simulink model "octocopter_control_flow"  (R2024a)
settings: Solver=FixedStepAuto  StartTime=0.0  StopTime=inf
model workspace (MAT data in the model file):
  Ixx_values = 1.545e-05
  Iyy_values = 0.00073574
  Izz_values = 0.00074861
  base_link_Ixx = 7.46
  base_link_Iyy = 1.52
  base_link_Izz = 8.88
  base_link_mass = 19.0939
  gps0_Ixx = 2.1733e-06
  gps0_Iyy = 2.1733e-06
  gps0_Izz = 1.8e-07
  gps0_mass = 0.01
  i = 8
  imu_link_Ixx = 1e-05
  imu_link_Iyy = 1e-05
  imu_link_Izz = 1e-05
  imu_link_mass = 0.015
  masses = 0.085251
  phi = sym
  phi.s = 'symobj::fromString("eJytVL1OwzAQdpqWPwkhoaJCp0jwBIydCoKBEYoYWCyHmGLkOCXnlGbjKXgneCpst6LONQ0MjfTJzt35u+/uLIeEkBYhH59mbYdBxyzDPpl/odl3F3sTQ3YtoAQGIMbKmSv+c4t3LvIkmrJcsFjySLGUQ1QATyKhIijTLH69KtK0vEm40uJZ8Jz4OVuIs23xksnE2HteTL9mj/W6syAzjexbFqATKWKXe48sv30L4HpUphdSMOAwr/PEy/HtxQeIe9tiAoI+MFvY8MzTebo84/79vAcWc02DwfVskpmO4Vl8efFt9N9BfE6Hx+P7QgujEfOv1EF/J13xHVmsHeWSs1M7jyIGpP2wQYebFeVvBZPkr3429crn3LGATE65uwGV3jjfJQPxNOIa8fRQrKsn51ZZhd/hjlZ6gTV1US2+77hulkJpPnYdXs31uLlcrv6caZGp+rpu6eYejP9epKZHofniCJXw2UpeVyQ1iZkC6j0sliP0mhFEixXbgzX2+8X6AxDlhOk=", 2)'
  phi.Digits = 32
  rotors(1).mass = 0.085251
  rotors(1).Ixx = 1.545e-05
  rotors(1).Iyy = 0.00073574
  rotors(1).Izz = 0.00074861
  rotors(2).mass = 0.085251
  rotors(2).Ixx = 1.545e-05
  rotors(2).Iyy = 0.00073574
  rotors(2).Izz = 0.00074861
  rotors(3).mass = 0.085251
  rotors(3).Ixx = 1.545e-05
  rotors(3).Iyy = 0.00073574
  rotors(3).Izz = 0.00074861
  rotors(4).mass = 0.085251
  rotors(4).Ixx = 1.545e-05
  rotors(4).Iyy = 0.00073574
  rotors(4).Izz = 0.00074861
  rotors(5).mass = 0.085251
  rotors(5).Ixx = 1.545e-05
  rotors(5).Iyy = 0.00073574
  rotors(5).Izz = 0.00074861
  rotors(6).mass = 0.085251
  rotors(6).Ixx = 1.545e-05
  rotors(6).Iyy = 0.00073574
  rotors(6).Izz = 0.00074861
  rotors(7).mass = 0.085251
  rotors(7).Ixx = 1.545e-05
  rotors(7).Iyy = 0.00073574
  rotors(7).Izz = 0.00074861
  rotors(8).mass = 0.085251
  rotors(8).Ixx = 1.545e-05
  rotors(8).Iyy = 0.00073574
  rotors(8).Izz = 0.00074861
  theta = sym
  theta.s = 'symobj::fromString("eJytVL1OwzAQdpqWPwkhoaJCp0jwBIydCoKBESoxsFgOOYqR45ScU5qNp+CdylNhuxV13DQwNNInO3fn7767sxwSQlqEfH7ptR0GHb0M+2TxhXrfXe51DNk3wBIZIh9La674Lw0+gOdJNGU5Z7GASLIUMCoQkojLCMs0i99uijQt7xKQir9wyImbs+Vxtg1eM5Foe8+J6dfsfb32LIpMefYdA1SJ4LHNfUBW36EBghqV6ZXgDAEXdZ45Ob6d+MDj3jWYIKePzBQ2vHB0nq/O2H8375HBQtNgcDubZLpj/izmTnzb++94fFaHw+P6QgOt0edfq4P+TrriOzHYOMoVZ6d2HkWMnvbjBh12VhTeCybIX/1s6pXLuWeAmZiCvQGV3ljfNUP+PALl8fS8WFtPDkZZhd/igVZ64WvqerW4vtO6WXKpYGw7vJ7raXu5bP05UzyT9XXd0+09GP+9SE2PQvPF4TKB2VpeWyTViZlE6jwshiN0mhFEy9W3BxvssFx/ABFthPo=", 2)'
  theta.Digits = 32
  total_Ixx = 7.46
  total_Iyy = 1.53
  total_Izz = 8.89
  total_mass = 20
  total_rotor_Ixx = 0.0001236
  total_rotor_Iyy = 0.00588592
  total_rotor_Izz = 0.00598888
  total_rotor_masses = 0.682008
  u = sym
  u.s = 'symobj::fromString("eJytVL1OwzAQdpqWPwkhoaJCp0jwBIydCoKBESoxsFgOOYqR45ScU5qNp+CdylNhuxV13DQwNNInO3fn7767sxwSQlqEfH7ptR0GHb0M+2TxhXrfXe51DNk3wBIZIh9La674Lw0+gOdJNGU5Z7GASLIUMCoQkojLCMs0i99uijQt7xKQir9wyImbs+Vxtg1eM5Foe8+J6dfsfb32LIpMefYdA1SJ4LHNfUBW36EBghqV6ZXgDAEXdZ45Ob6d+MDj3jWYIKePzBQ2vHB0nq/O2H8375HBQtNgcDubZLpj/izmTnzb++94fFaHw+P6QgOt0edfq4P+TrriOzHYOMoVZ6d2HkWMnvbjBh12VhTeCybIX/1s6pXLuWeAmZiCvQGV3ljfNUP+PALl8fS8WFtPDkZZhd/igVZ64WvqerW4vtO6WXKpYGw7vJ7raXu5bP05UzyT9XXd0+09GP+9SE2PQvPF4TKB2VpeWyTViZlE6jwshiN0mhFEy9W3Bxvs0+X6AxH1hQs=", 2)'
  u.Digits = 32
  v = sym
  v.s = 'symobj::fromString("eJytVL1OwzAQdpqWPwkhoaJCp0jwBIydCoKBESoxsFgOOYqR45ScU5qNjTfgneCpsN2KOm4aGBrpk52783ff3VkOCSEtQt4/9doOg45ehn0y/0K97y72OobsGmCJDJGPpTVX/OcGb8DzJJqynLNYQCRZChgVCEnEZYRlmsUvV0WaljcJSMWfOOTEzdnyONsGz5lItL3nxPRr9r5eexZFpjz7lgGqRPDY5t4jy2/fAEGNyvRCcIaA8zpPnBzfTnzgcW8bTJDTe2YKG545Ok+XZ+y/m/fAYK5pMLieTTLdMX8WX0582/vveHxWh8Pj+kIDrdHnX6mD/k664jsyWDvKJWendh5FjJ72wwYddlYUXgsmyF/9bOqVy7ljgJmYgr0Bld5Y3yVD/jgC5fH0vFhbTw5GWYXf4o5WeuFr6nq1uL7jullyqWBsO7ya62FzuWz9OVM8k/V13dLNPRj/vUhNj0LzxeEygdlKXlsk1YmZROo8LIYjdJoRRIvVtwdr7B+L9QcSfYUc", 2)'
  v.Digits = 32
  w = sym
  w.s = 'symobj::fromString("eJytVL1OwzAQdpqWPwkhoaJCp0jwBIydCoKBESoxsFgOOYqR45ScU5qNp0C8EjwVtltRx00DQyN9snN3/u67O8shIaRFyPuHXtth0NHLsE/mX6j33cVex5BdAyyRIfKxtOaK/9zgDXieRFOWcxYLiCRLAaMCIYm4jLBMs/jlqkjT8iYBqfgTh5y4OVseZ9vgOROJtvecmH7N3tdrz6LIlGffMkCVCB7b3Htk+e0bIKhRmV4IzhBwXueJk+PbiQ887m2DCXJ6z0xhwzNH5+nyjP138x4YzDUNBtezSaY75s/iy4lve/8dj8/qcHhcX2igNfr8K3XQ30lXfEcGa0e55OzUzqOI0dN+2KDDzorCa8EE+aufTb1yOXcMMBNTsDeg0hvru2TIH0egPJ6eF2vrycEoq/Bb3NFKL3xNXa8W13dcN0suFYxth1dzPWwul60/Z4pnsr6uW7q5B+O/F6npUWi+OFwmMFvJa4ukOjGTSJ2HxXCETjOCaLH69mCN/XOx/gATBYUt", 2)'
  w.Digits = 32
  x = sym
  x.s = 'symobj::fromString("eJytVEtOwzAQdZqWn4SQUFGhq0hwApZdFQQLllCJBRvLIUMxcpyScUqz4xTcgaPAqbDdijpuGlg00pOdmfGbNzOWQ0JIi5D3D722w6Cjl2GfzL9Q77uLvY4huwZYIkPkY2nNFf+5wRvwPImmLOcsFhBJlgJGBUIScRlhmWbxy1WRpuVNAlLxJw45cXO2PM62wXMmEm3vOTH9mr2v155FkSnPvmWAKhE8trn3yPLbN0BQozK9EJwh4LzOEyfHtxMfeNzbBhPk9J6ZwoZnjs7T5Rn77+Y9MJhrGgyuZ5NMd8yfxZcT3/b+Ox6f1eHwuL7QQGv0+VfqoL+TrviODNaOcsnZqZ1HEaOn/bBBh50VhdeCCfJXP5t65XLuGGAmpmBvQKU31nfJkD+OQHk8PS/W1pODUVbht7ijlV74mrpeLa7vuG6WXCoY2w6v5nrYXC5bf84Uz2R9Xbd0cw/Gfy9S06PQfHG4TGC2ktcWSXViJpE6D4vhCJ1mBNFi9e3BGvvnYv0BE42FPg==", 2)'
  x.Digits = 32
  y = sym
  y.s = 'symobj::fromString("eJytVEtOwzAQdZqWn4SQUFGhq0hwApZdFQQLllCJBRvLIUMxcpyScUqz4xQchhvAqbDdijpuGlg00pOdmfGbNzOWQ0JIi5D3D722w6Cjl2GfzL9Q77uLvY4huwZYIkPkY2nNFf+5wRvwPImmLOcsFhBJlgJGBUIScRlhmWbxy1WRpuVNAlLxJw45cXO2PM62wXMmEm3vOTH9mr2v155FkSnPvmWAKhE8trn3yPLbN0BQozK9EJwh4LzOEyfHtxMfeNzbBhPk9J6ZwoZnjs7T5Rn77+Y9MJhrGgyuZ5NMd8yfxZcT3/b+Ox6f1eHwuL7QQGv0+VfqoL+TrviODNaOcsnZqZ1HEaOn/bBBh50VhdeCCfJXP5t65XLuGGAmpmBvQKU31nfJkD+OQHk8PS/W1pODUVbht7ijlV74mrpeLa7vuG6WXCoY2w6v5nrYXC5bf84Uz2R9Xbd0cw/Gfy9S06PQfHG4TGC2ktcWSXViJpE6D4vhCJ1mBNFi9e3BGvvnYv0BFBWFTw==", 2)'
  y.Digits = 32
  z = sym
  z.s = 'symobj::fromString("eJytVL1OwzAQdpqWPwkhoaJCp0jwBIydCoKBESoxsFgOOYqR45ScU5qNp+CdgJfCdivquGlgaKRPdu7O3313ZzkkhLQIef/QazsMOnoZ9sn8C/W+u9jrGLJrgCUyRD6W1lzxnxu8Ac+TaMpyzmIBkWQpYFQgJBGXEZZpFr9cFWla3iQgFX/ikBM3Z8vjbBs8ZyLR9p4T06/Z+3rtWRSZ8uxbBqgSwWObe48sv30DBDUq0wvBGQLO6zxxcnw58YHHvW0wQU7vmSlseOboPF2esf9u3gODuabB4Ho2yXTH/Fl8OvFt77/j8VkdDo/rCw20Rp9/pQ76O+mK78hg7SiXnJ3aeRQxetoPG3TYWVF4LZggf/WzqVcu544BZmIK9gZUemN9lwz54wiUx9PzYm09ORhlFX6LO1rpha+p69Xi+o7rZsmlgrHt8Gquh83lsvXnTPFM1td1Szf3YPz3IjU9Cs0Xh8sEZit5bZFUJ2YSqfOwGI7QaUYQLVbfHqyxfy/WHxSdhWA=", 2)'
  z.Digits = 32
values from neighbouring files (symbols this model uses):
  err1Enable = 0    [drone_6dof.m]    (also in octocopter_model_for_agressive.m; octocopter_model_for_orbit.m)
  err2Enable = 0    [drone_6dof.m]    (also in octocopter_model_for_agressive.m; octocopter_model_for_orbit.m)
  err3Enable = 0    [drone_6dof.m]    (also in octocopter_model_for_agressive.m; octocopter_model_for_orbit.m)
  err4Enable = 0    [drone_6dof.m]    (also in octocopter_model_for_agressive.m; octocopter_model_for_orbit.m)
  err5Enable = 0    [drone_6dof.m]    (also in octocopter_model_for_agressive.m; octocopter_model_for_orbit.m)
  err6Enable = 0    [drone_6dof.m]    (also in octocopter_model_for_agressive.m; octocopter_model_for_orbit.m)
  err7Enable = 0    [drone_6dof.m]    (also in octocopter_model_for_agressive.m; octocopter_model_for_orbit.m)
  err8Enable = 0    [drone_6dof.m]    (also in octocopter_model_for_agressive.m; octocopter_model_for_orbit.m)
  EulerInt_initial = [0;0;0]    [drone_6dof.m]    (also in octocopter_model_for_agressive.m; octocopter_model_for_orbit.m)
  motorErr1Time = 0    [drone_6dof.m]    (also in octocopter_model_for_agressive.m; octocopter_model_for_orbit.m)
  motorErr2Time = 0    [drone_6dof.m]    (also in octocopter_model_for_agressive.m; octocopter_model_for_orbit.m)
  motorErr3Time = 0    [drone_6dof.m]    (also in octocopter_model_for_agressive.m; octocopter_model_for_orbit.m)
  motorErr4Time = 0    [drone_6dof.m]    (also in octocopter_model_for_agressive.m; octocopter_model_for_orbit.m)
  motorErr5Time = 0    [drone_6dof.m]    (also in octocopter_model_for_agressive.m; octocopter_model_for_orbit.m)
  motorErr6Time = 0    [drone_6dof.m]    (also in octocopter_model_for_agressive.m; octocopter_model_for_orbit.m)
  motorErr7Time = 0    [drone_6dof.m]    (also in octocopter_model_for_agressive.m; octocopter_model_for_orbit.m)
  motorErr8Time = 0    [drone_6dof.m]    (also in octocopter_model_for_agressive.m; octocopter_model_for_orbit.m)
  omegaInt_initial = [0;0;0]    [drone_6dof.m]    (also in octocopter_model_for_agressive.m; octocopter_model_for_orbit.m)
  PosInertialInt_initial = [0;0;0]    [drone_6dof.m]    (also in octocopter_model_for_agressive.m; octocopter_model_for_orbit.m)
  vbInt_initial = [0;0;0]    [drone_6dof.m]    (also in octocopter_model_for_agressive.m; octocopter_model_for_orbit.m)
undefined symbols (not defined in the file or in its folder): DiscIntNeverNeededParam, PID_x_D, PID_x_I, PID_x_N, PID_y_D, PID_y_I, PID_y_N, PID_z_D, PID_z_I, PID_z_N, rad, rotor_max_rad_per_s, rotor_min_rad_per_s, s
libraries: robotlib x15, slpidlib x10, aerolibconvert2 x10, cstblocks x7, simulink x6, sharedtransform x4, dspmathops x1, vrlib x1, sharedutil x1, simulink_extras x1
(part 1 of 2)
settings Model: PacingRate=10  Creator=hmcl  LastModifiedBy=hmcl
settings RTWCC: GPUComputeCapability=3.5

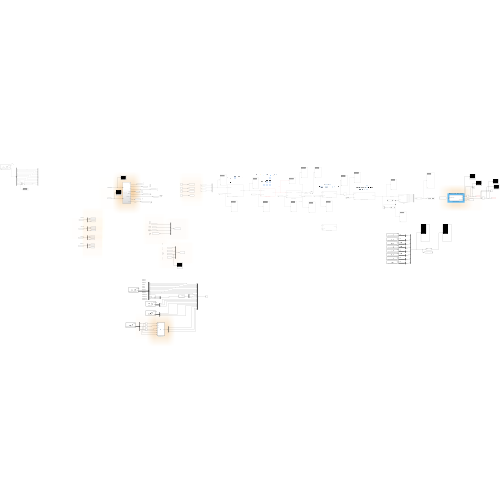
[thumbnail: Simulink's stored preview of the top-level diagram]
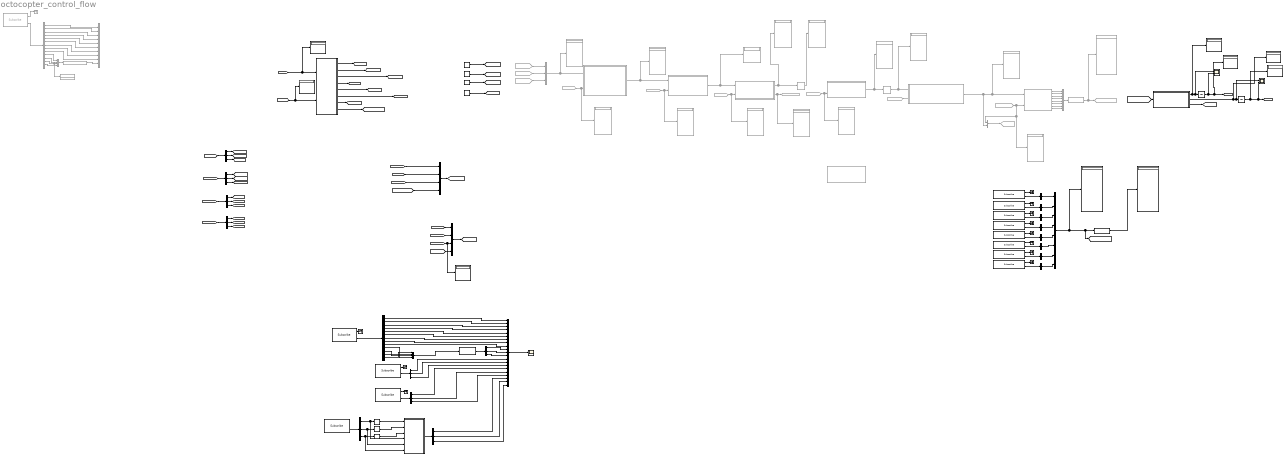
== system octocopter_control_flow ==
  note: Position.X,
      | Position.Y,
      | Position.Z,
      | Linear.X
      | Linear.Y
      | Linear.Z
      | Angular.X
      | Angular.Y
      | Angular.Z
      | Orientation.X,
      | Orientation.Y,
      | Orientation.Z,
      | Orientation.W,
  note: earth frame
  note: phi_dot
      | theta_dot
      | psi_dot
  note: x_dot
      | y_dot
      | z_dot
  note: phi
      | theta
      | psi
  note: u
      | v
      | w
  note: p
      | q
      | r
  note: p_dot
      | q_dot
      | r_dot
  note: u_dot
      | v_dot
      | w_dot
  note: x
      | y
      | z
  note: earth frame
  note: earth frame
  note: earth frame
  note: Motor Force and Torque
  note: u_dot
      | v_dot
      | w_dot
  note: x_dot
      | y_dot
      | z_dot
  note: phi_dot
      | theta_dot
      | psi_dot
  note: p_dot
      | q_dot
      | r_dot
  note: phi
      | theta
      | psi
  note: p
      | q
      | r
  note: x
      | y
      | z
  note: u
      | v
      | w
  Angular Rate Controller : Subsystem  Commented=on  mask{MC_ROLLRATE_K=0.01, MC_ROLLRATE_P=0.044, MC_ROLLRATE_I=0.05, MC_ROLLRATE_D=0.0012, MC_RR_INT_LIM=1000, MC_PITCHRATE_K=0.01, MC_PITCHRATE_P=0.044, MC_PITCHRATE_I=0.05, MC_PITCHRATE_D=0.0012, MC_PR_INT_LIM=1000, MC_YAWRATE_K=0.01, MC_YAWRATE_P=0.044, MC_YAWRATE_I=0.05, MC_YAWRATE_D=0.0012, MC_YR_INT_LIM=1000, IMU_DGYRO_CUTOFF=30, IMU_GYRO_CUTOFF=40}
      mask prompts: MC_ROLLRATE_K "MC_ROLLRATE_K ="; MC_ROLLRATE_P "MC_ROLLRATE_P ="; MC_ROLLRATE_I "MC_ROLLRATE_I ="; MC_ROLLRATE_D "MC_ROLLRATE_D ="; MC_RR_INT_LIM "MC_RR_INT_LIM ="; MC_PITCHRATE_K "MC_PITCHRATE_K ="; MC_PITCHRATE_P "MC_PITCHRATE_P ="; MC_PITCHRATE_I "MC_PITCHRATE_I ="; MC_PITCHRATE_D "MC_PITCHRATE_D ="; MC_PR_INT_LIM "MC_PR_INT_LIM ="; MC_YAWRATE_K "MC_YAWRATE_K ="; MC_YAWRATE_P "MC_YAWRATE_P ="; MC_YAWRATE_I "MC_YAWRATE_I ="; MC_YAWRATE_D "MC_YAWRATE_D ="; MC_YR_INT_LIM "MC_YR_INT_LIM ="; IMU_DGYRO_CUTOFF "IMU_DGYRO_CUTOFF ="; IMU_GYRO_CUTOFF "IMU_GYRO_CUTOFF ="
      mask DialogControl DescTextVar Prompt: Angular rate controller, based on PX4 architecture
      mask DialogControl ROLL Prompt: Roll
      mask DialogControl PITCH Prompt: Pitch
      mask DialogControl YAW Prompt: Yaw
  Angular Velocity Conversion : aerolibconvert2/Angular Velocity Conversion  Commented=on  IU=rad/s  OU=rpm
  Angular Velocity Conversion1 : aerolibconvert2/Angular Velocity Conversion  IU=rad/s  OU=rpm
  Attitude Controller : Subsystem  Commented=on  mask{MC_ROLL_P=4, MC_PITCH_P=4, MC_YAW_P=4, MC_ROLLRATE_MAX=10, MC_PITCHRATE_MAX=10, MC_YAWRATE_MAX=10, MC_ACRO_R_MAX=2, MC_YAW_WEIGHT=0.1}
      mask prompts: MC_ROLL_P "MC_ROLL_P ="; MC_PITCH_P "MC_PITCH_P ="; MC_YAW_P "MC_YAW_P ="; MC_ROLLRATE_MAX "MC_ROLLRATE_MAX ="; MC_PITCHRATE_MAX "MC_PITCHRATE_MAX ="; MC_YAWRATE_MAX "MC_YAWRATE_MAX ="; MC_ACRO_R_MAX "MC_ACRO_R_MAX ="; MC_YAW_WEIGHT "MC_YAW_WEIGHT ="
      mask DialogControl DescTextVar Prompt: Attitude Controller - based on PX4 architecture
  Attitude Controller1 : Subsystem  Commented=on  mask{MC_ROLL_P=6.5, MC_PITCH_P=6.5, MC_YAW_P=2.8, MC_ROLLRATE_MAX=220, MC_PITCHRATE_MAX=220, MC_YAWRATE_MAX=200, MC_ACRO_R_MAX=100, MC_YAW_WEIGHT=0.4}
      mask prompts: MC_ROLL_P "MC_ROLL_P ="; MC_PITCH_P "MC_PITCH_P ="; MC_YAW_P "MC_YAW_P ="; MC_ROLLRATE_MAX "MC_ROLLRATE_MAX ="; MC_PITCHRATE_MAX "MC_PITCHRATE_MAX ="; MC_YAWRATE_MAX "MC_YAWRATE_MAX ="; MC_ACRO_R_MAX "MC_ACRO_R_MAX ="; MC_YAW_WEIGHT "MC_YAW_WEIGHT ="
      mask DialogControl DescTextVar Prompt: Attitude Controller - based on PX4 architecture
  Bus Selector{,3..9} (8 alike) : BusSelector  OutputSignals=Data
  Bus Selector1 : BusSelector  OutputSignals=Pose.Pose.Position.X,Pose.Pose.Position.Y,Pose.Pose.Position.Z,Twist.Twist.Linear.X,Twist.Twist.Linear.Y,Twist.Twist.Linear.Z,Twist.Twist.Angular.X,Twist.Twist.Angular.Y,Twist.Twist.Angular.Z,Pose.Pose.Orientation.X,Pose.Pose.Orientation.Y,Pose.Pose.Orientation.Z,Pose.Pose.Orientation.W
  Bus Selector10 : BusSelector  OutputSignals=X,Y,Z
  Bus Selector11 : BusSelector  OutputSignals=X,Y,Z
  Bus Selector12 : BusSelector  OutputSignals=Twist.Twist.Angular.X,Twist.Twist.Angular.Y,Twist.Twist.Angular.Z
  Bus Selector2 : BusSelector  Commented=on  OutputSignals=Pose.Pose.Position.X,Pose.Pose.Position.Y,Pose.Pose.Position.Z,Twist.Twist.Linear.X,Twist.Twist.Linear.Y,Twist.Twist.Linear.Z,Twist.Twist.Angular.X,Twist.Twist.Angular.Y,Twist.Twist.Angular.Z,Pose.Pose.Orientation.X,Pose.Pose.Orientation.Y,Pose.Pose.Orientation.Z,Pose.Pose.Orientation.W
  Constant : Constant  Value=0
  Constant1 : Constant  Value=0
  Constant2 : Constant  Value=10
  Constant3 : Constant  Value=0
  ControlMatrixAllocation Mixer : Subsystem  Commented=on  mask{Ct=5.781e-06, Cq=1.839e-07, L1=0.545, L2=0.36, L3=1.08}
      mask prompts: Ct "Ct ="; Cq "Cq ="; L1 "L1 ="; L2 "L2 ="; L3 "L3 ="
  Demux{,1..5} (6 alike) : Demux  Outputs=3
  Derivative : Derivative
  Derivative1 : Derivative
  Derivative2 : Derivative
  Display{,1..2,10,12..23} (16 alike) : Display  Commented=on
  Display{3..9,24..25} (9 alike) : Display
  From : From  Commented=on  GotoTag=zRef
  From1 : From  Commented=on  GotoTag=yRef
  From10 : From  Commented=on  GotoTag=phithetapsi
  From11 : From  Commented=on  GotoTag=OMEGA
  From12 : From  Commented=on  GotoTag=desired_Thrust
  From2 : From  Commented=on  GotoTag=xRef
  From7 : From  Commented=on  GotoTag=xyz
  From8 : From  Commented=on  GotoTag=V
  From9 : From  Commented=on  GotoTag=desired_yaw
  Goto13 : Goto  Commented=on  GotoTag=desired_Thrust
  Goto25 : Goto  Commented=on  GotoTag=omegaMotorSpeed
  Goto32 : Goto  Commented=on  GotoTag=desired_input
  Inertial to Body : Subsystem  Commented=on  mask{m=total_mass}
      mask prompts: m "m ="
      mask DialogControl DescTextVar Prompt: Acceleration and yaw to attitude Controller - based on PX4 architecture
  MATLAB Function : MATLAB Function  TreatAsAtomicUnit=on
  MotorForceCalculation : Subsystem  mask{Ct=6.5, Cq=-0.325, L1=0.545, L2=0.36, L3=1.08}
      mask prompts: Ct "Ct ="; Cq "Cq ="; L1 "L1 ="; L2 "L2 ="; L3 "L3 ="
  Mux : Mux  Commented=on  Inputs=3
  Mux1 : Mux  Commented=on  Inputs=8
  Mux2 : Mux  Commented=on  Inputs=10
  Mux3 : Mux
  Mux4 : Mux
  Mux5 : Mux  Inputs=21
  Mux6 : Mux  Commented=on
  Mux7 : Mux
  Mux8 : Mux  Commented=on  Inputs=2
  Mux9 : Mux  Inputs=8
  Position Controller : Subsystem  Commented=on  mask{MPC_XY_P=1, MPC_XY_VEL_ALL=10, MPC_Z_P=1, MPC_Z_VEL_ALL=100}
      mask prompts: MPC_XY_P "MPC_XY_P ="; MPC_XY_VEL_ALL "MPC_XY_VEL_ALL ="; MPC_Z_P "MPC_Z_P ="; MPC_Z_VEL_ALL "MPC_Z_VEL_ALL ="
      mask DialogControl DescTextVar Prompt: Position Controller - based on PX4 architecture
  Quaternions to Rodrigues1 : Quat2Rod  Commented=on
  Quaternions to Rotation Angles : sharedtransform/Quaternions to Rotation Angles  rotationOrder=ZYX  aMode=aMode
  Rate Transition2 : RateTransition  Commented=on  OutPortSampleTime=1/1000
  Rate Transition5 : RateTransition  Commented=on  OutPortSampleTime=1/1000
  Scope : Scope  NumInputPorts=2
  Scope1 : Scope  NumInputPorts=2
  Scope2 : Scope
  Subscribe : robotlib/Subscribe  topicSource=Select from ROS network  topic=/my/octocopter3/motor_speed/0  messageType=std_msgs/Float64  SampleTime=-1  legacyBusStruct=off  messageQueueLength=1
  Subscribe1 : robotlib/Subscribe  topicSource=Select from ROS network  topic=/mavros/local_position/odom  messageType=nav_msgs/Odometry  SampleTime=-1  legacyBusStruct=off  messageQueueLength=1
  Subscribe10 : robotlib/Subscribe  topicSource=Select from ROS network  topic=/thrust_vector  messageType=geometry_msgs/Vector3  SampleTime=-1  legacyBusStruct=off  messageQueueLength=1
  Subscribe11 : robotlib/Subscribe  topicSource=Select from ROS network  topic=/torque_vector  messageType=geometry_msgs/Vector3  SampleTime=-1  legacyBusStruct=off  messageQueueLength=1
  Subscribe12 : robotlib/Subscribe  topicSource=Select from ROS network  topic=/mavros/local_position/odom  messageType=nav_msgs/Odometry  SampleTime=-1  legacyBusStruct=off  messageQueueLength=1
  Subscribe2 : robotlib/Subscribe  Commented=on  topicSource=Select from ROS network  topic=/mavros/local_position/odom  messageType=nav_msgs/Odometry  SampleTime=-1  legacyBusStruct=off  messageQueueLength=1
  Subscribe3 : robotlib/Subscribe  topicSource=Select from ROS network  topic=/my/octocopter3/motor_speed/1  messageType=std_msgs/Float64  SampleTime=-1  legacyBusStruct=off  messageQueueLength=1
  Subscribe4 : robotlib/Subscribe  topicSource=Select from ROS network  topic=/my/octocopter3/motor_speed/2  messageType=std_msgs/Float64  SampleTime=-1  legacyBusStruct=off  messageQueueLength=1
  Subscribe5 : robotlib/Subscribe  topicSource=Select from ROS network  topic=/my/octocopter3/motor_speed/3  messageType=std_msgs/Float64  SampleTime=-1  legacyBusStruct=off  messageQueueLength=1
  Subscribe6 : robotlib/Subscribe  topicSource=Select from ROS network  topic=/my/octocopter3/motor_speed/4  messageType=std_msgs/Float64  SampleTime=-1  legacyBusStruct=off  messageQueueLength=1
  Subscribe7 : robotlib/Subscribe  topicSource=Select from ROS network  topic=/my/octocopter3/motor_speed/5  messageType=std_msgs/Float64  SampleTime=-1  legacyBusStruct=off  messageQueueLength=1
  Subscribe8 : robotlib/Subscribe  topicSource=Select from ROS network  topic=/my/octocopter3/motor_speed/6  messageType=std_msgs/Float64  SampleTime=-1  legacyBusStruct=off  messageQueueLength=1
  Subscribe9 : robotlib/Subscribe  topicSource=Select from ROS network  topic=/my/octocopter3/motor_speed/7  messageType=std_msgs/Float64  SampleTime=-1  legacyBusStruct=off  messageQueueLength=1
  Subsystem : Subsystem
  Terminator{,1..10} (11 alike) : Terminator
  Terminator12 : Terminator  Commented=on
  Unit Delay : UnitDelay  SampleTime=-1  HasFrameUpgradeWarning=on
  Unit Delay1 : UnitDelay  SampleTime=-1  HasFrameUpgradeWarning=on
  Velocity Controller : Subsystem  Commented=on  mask{MPC_XY_VEL_P_ACC=1, MPC_XY_VEL_I_ACC=0.1, MPC_XY_VEL_D_ACC=0.01, MPC_Z_VEL_P_ACC=1, MPC_Z_VEL_I_ACC=0.1, MPC_Z_VEL_D_ACC=0.01, MPC_VELD_LP=5.0, MPC_TILTMAX_AIR=45, MPC_THR_MAX=1000}
      mask prompts: MPC_XY_VEL_P_ACC "MPC_XY_VEL_P_ACC ="; MPC_XY_VEL_I_ACC "MPC_XY_VEL_I_ACC ="; MPC_XY_VEL_D_ACC "MPC_XY_VEL_D_ACC ="; MPC_Z_VEL_P_ACC "MPC_Z_VEL_P_ACC ="; MPC_Z_VEL_I_ACC "MPC_Z_VEL_I_ACC ="; MPC_Z_VEL_D_ACC "MPC_Z_VEL_D_ACC ="; MPC_VELD_LP "MPC_VELD_LP ="; MPC_TILTMAX_AIR "MPC_TILTMAX_AIR ="; MPC_THR_MAX "MPC_THR_MAX ="
      mask DialogControl DescTextVar Prompt: Velocity Controller - based on PX4 architecture
      mask DialogControl Container3 Prompt: XY -  Velocity
      mask DialogControl Container4 Prompt: Z - Velocity
      mask DialogControl Container5 Prompt: General Parameters
  wires:
  Quaternions to Rodrigues1/1 -> Mux2/10
  Bus Selector2/4 -> Mux2/4  "<X>"
  Bus Selector2/10 -> Mux6/1  "<X>"
  Bus Selector2/3 -> Mux2/3  "<Z>"
  Bus Selector2/7 -> Mux2/7  "<X>"
  Bus Selector2/8 -> Mux2/8  "<Y>"
  Bus Selector2/1 -> Mux2/1  "<X>"
  Bus Selector2/9 -> Mux2/9  "<Z>"
  Mux6/1 -> Quaternions to Rodrigues1/1
  Subscribe2/2 -> Bus Selector2/1
  Bus Selector2/6 -> Mux2/6  "<Z>"
  Bus Selector2/12 -> Mux6/3, Display1/1  "<Z>"
  Bus Selector2/11 -> Mux6/2  "<Y>"
  Bus Selector2/5 -> Mux2/5  "<Y>"
  Bus Selector2/2 -> Mux2/2  "<Y>"
  Bus Selector2/13 -> Mux6/4  "<W>"
  Subscribe2/1 -> Terminator12/1
  Subsystem/1(xyz) -> [xyz]
  Subsystem/2(V) -> [V]  "V"
  Subsystem/4(VB_dot) -> [VB_dot]  "VB_dot"
  Subsystem/5(phithetapsi) -> [phithetapsi]
  Subsystem/8(pqr_dot) -> [OMEGAB_dot]  "pqr_dot"
  Subsystem/7(pqr) -> [OMEGAB]  "pqr"
  Subsystem/3(VB) -> [VB]  "VB"
  Subsystem/6(phithetapsi_dot) -> [OMEGA]
  [xyz] -> Demux/1
  [V] -> Demux1/1
  [phithetapsi] -> Demux2/1
  [OMEGA] -> Demux3/1
  Demux2/1 -> [phi]
  Demux2/2 -> [theta]
  Demux2/3 -> [psi]
  Demux3/1 -> [phidot]
  Demux3/2 -> [thetadot]
  Demux3/3 -> [psidot]
  Demux/3 -> [z]
  Demux/1 -> [x]
  Demux/2 -> [y]
  Demux1/1 -> [x_dot]
  Demux1/2 -> [y_dot]
  Demux1/3 -> [z_dot]
  From7/1 -> Display13/1, Position Controller/2(Current position)  "xyz"
  From2/1 -> Mux/1
  From1/1 -> Mux/2
  From/1 -> Mux/3
  Mux/1 -> Display12/1, Position Controller/1(Setpoint position)
  Velocity Controller/1(Acc S.P) -> Display2/1, Inertial to Body/1(Setpoints acceleration)  "Acc S.P"
  From9/1 -> Display15/1, Inertial to Body/2(Yaw.SP)
  Inertial to Body/1(quat_attitude_sp) -> Display16/1, Rate Transition2/1  "attitude qutanion value"
  Inertial to Body/2(Thrust) -> Display22/1, Goto13/1  "desired thrust"
  Rate Transition2/1 -> Display17/1
  From10/1 -> Display23/1, Attitude Controller/2(Orientation)  "phithetapsi"
  Attitude Controller/1(S.P Rates) -> Display18/1, Rate Transition5/1  "S.P Rates"
  Rate Transition5/1 -> Display19/1, Angular Rate Controller/1(rates s.p)
  From11/1 -> Angular Rate Controller/2(Gyro)
  Angular Rate Controller/1(Delta S.P) -> Mux8/2, Display20/1, ControlMatrixAllocation Mixer/1(Tau_roll,pitch,yaw)  "desired_torque"
  From12/1 -> Mux8/1, Display21/1, ControlMatrixAllocation Mixer/2(Thrust)  "desire_thrust"
  Constant/1 -> [xRef]
  Constant2/1 -> [zRef]
  Constant1/1 -> [yRef]
  Constant3/1 -> [desired_yaw]
  ControlMatrixAllocation Mixer/1(Omega 1) -> Mux1/1
  ControlMatrixAllocation Mixer/2(Omega 2) -> Mux1/2
  ControlMatrixAllocation Mixer/3(Omega 3) -> Mux1/3
  ControlMatrixAllocation Mixer/4(Omega 4) -> Mux1/4
  ControlMatrixAllocation Mixer/5(Omega 5) -> Mux1/5
  ControlMatrixAllocation Mixer/6(Omega 6) -> Mux1/6
  ControlMatrixAllocation Mixer/7(Omega 7) -> Mux1/7
  ControlMatrixAllocation Mixer/8(Omega 8) -> Mux1/8
  Mux1/1 -> Angular Velocity Conversion/1
  MotorForceCalculation/1(FB) -> Display8/1, Scope/1, Unit Delay/1
  MotorForceCalculation/2(MB) -> Display9/1, Scope1/1, Unit Delay1/1
  [omegaMotorSpeed] -> MotorForceCalculation/1(omegaMotorSpeed)
  [FB] -> Display4/1, Subsystem/1(FB)
  [MB] -> Display5/1, Subsystem/2(MB)
  From8/1 -> Display/1, Velocity Controller/2(current velocity)
  Position Controller/1(desired vel) -> Display14/1, Velocity Controller/1(Setpoint velocity)  "V_sp"
  Unit Delay/1 -> Scope/2, [FB], Display6/1  "FB"
  Unit Delay1/1 -> Display7/1, [MB], Scope1/2  "MB"
  [V] -> Mux3/1
  [VB_dot] -> Mux3/2
  Mux3/1 -> [state_X_dot]
  MotorForceCalculation/3(desired_input) -> [desired_input]  "desired_input"
  [OMEGA] -> Mux3/3
  [OMEGAB_dot] -> Mux3/4
  Angular Velocity Conversion/1 -> Display10/1, Goto25/1  "Motor 1 - cmd"
  [xyz] -> Mux4/1
  [VB] -> Mux4/2
  [phithetapsi] -> Display3/1, Mux4/3
  [OMEGAB] -> Mux4/4
  Mux4/1 -> [state_x]
  Bus Selector1/2 -> Mux5/2  "<Y>"
  Bus Selector1/6 -> Mux5/6  "<Z>"
  Mux7/1 -> Quaternions to Rotation Angles/1
  Bus Selector1/7 -> Mux5/7  "<X>"
  Bus Selector1/9 -> Mux5/9  "<Z>"
  Bus Selector1/5 -> Mux5/5  "<Y>"
  Subscribe1/2 -> Bus Selector1/1
  Bus Selector1/1 -> Mux5/1  "<X>"
  Bus Selector1/3 -> Mux5/3  "<Z>"
  Bus Selector1/4 -> Mux5/4  "<X>"
  Subscribe1/1 -> Terminator1/1
  Bus Selector1/8 -> Mux5/8  "<Y>"
  Mux8/1 -> Goto32/1  "desired_input"
  Subscribe/1 -> Terminator/1
  Subscribe3/1 -> Terminator2/1
  Subscribe4/1 -> Terminator3/1
  Subscribe5/1 -> Terminator4/1
  Subscribe6/1 -> Terminator5/1
  Subscribe7/1 -> Terminator6/1
  Subscribe8/1 -> Terminator7/1
  Subscribe9/1 -> Terminator8/1
  Subscribe/2 -> Bus Selector/1
  Subscribe3/2 -> Bus Selector3/1
  Subscribe4/2 -> Bus Selector4/1
  Subscribe5/2 -> Bus Selector5/1
  Subscribe6/2 -> Bus Selector6/1
  Subscribe7/2 -> Bus Selector7/1
  Subscribe8/2 -> Bus Selector8/1
  Subscribe9/2 -> Bus Selector9/1
  Mux9/1 -> Display25/1, [omegaMotorSpeed], Angular Velocity Conversion1/1
  Bus Selector/1 -> Mux9/1  "<Data>"
  Bus Selector3/1 -> Mux9/2  "<Data>"
  Bus Selector4/1 -> Mux9/3  "<Data>"
  Bus Selector5/1 -> Mux9/4  "<Data>"
  Bus Selector6/1 -> Mux9/5  "<Data>"
  Bus Selector7/1 -> Mux9/6  "<Data>"
  Bus Selector8/1 -> Mux9/7  "<Data>"
  Bus Selector9/1 -> Mux9/8  "<Data>"
  Angular Velocity Conversion1/1 -> Display24/1
  Bus Selector1/13 -> Mux7/1  "<W>"
  Bus Selector1/12 -> Mux7/2  "<Z>"
  Bus Selector1/11 -> Mux7/3  "<Y>"
  Bus Selector1/10 -> Mux7/4  "<X>"
  Mux5/1 -> Scope2/1
  Quaternions to Rotation Angles/1 -> Demux4/1
  Demux4/1 -> Mux5/10
  Demux4/2 -> Mux5/11
  Demux4/3 -> Mux5/12
  Subscribe10/1 -> Terminator9/1
  Subscribe11/1 -> Terminator10/1
  Subscribe10/2 -> Bus Selector10/1
  Subscribe11/2 -> Bus Selector11/1
  Bus Selector11/1 -> Mux5/13  "<X>"
  Bus Selector11/2 -> Mux5/14  "<Y>"
  Bus Selector11/3 -> Mux5/15  "<Z>"
  Bus Selector10/1 -> Mux5/16  "<X>"
  Bus Selector10/2 -> Mux5/17  "<Y>"
  Bus Selector10/3 -> Mux5/18  "<Z>"
  Subscribe12/2 -> Bus Selector12/1
  Bus Selector12/1 -> MATLAB Function/4(p), Derivative/1  "<X>"
  Bus Selector12/2 -> MATLAB Function/5(q), Derivative1/1  "<Y>"
  Bus Selector12/3 -> Derivative2/1, MATLAB Function/6(r)  "<Z>"
  Derivative/1 -> MATLAB Function/1(p_dot)
  Derivative1/1 -> MATLAB Function/2(q_dot)
  Derivative2/1 -> MATLAB Function/3(r_dot)
  MATLAB Function/1(M_B) -> Demux5/1
  Demux5/1 -> Mux5/19
  Demux5/2 -> Mux5/20
  Demux5/3 -> Mux5/21

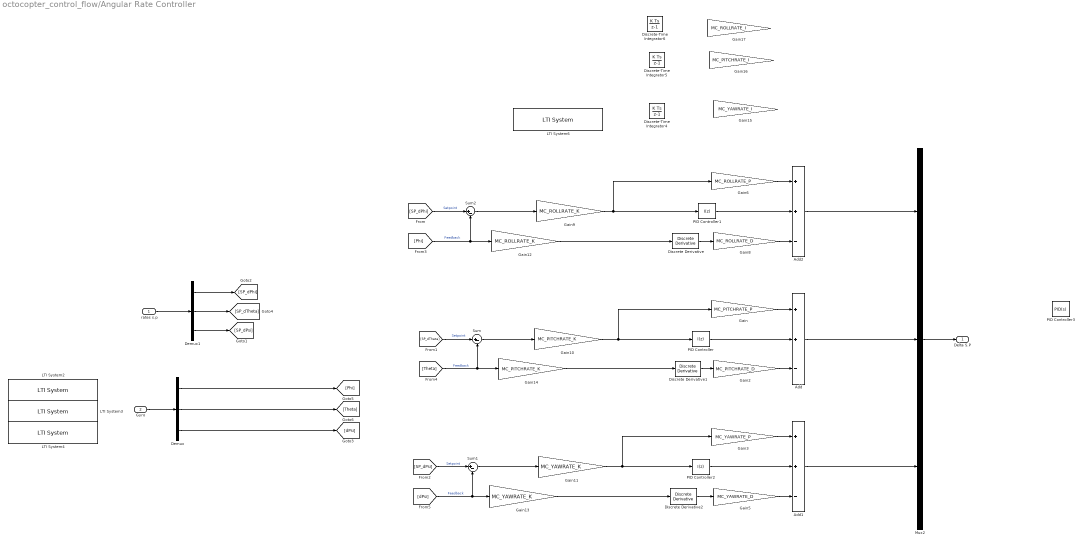
== system octocopter_control_flow/Angular Rate Controller ==
  rates s.p : Inport
  Gyro : Inport  Port=2
  Add : Sum  Inputs=++-
  Add1 : Sum  Inputs=++-
  Add2 : Sum  Inputs=++-
  Demux : Demux  Outputs=3
  Demux1 : Demux  Outputs=3
  Discrete Derivative : simulink/Discrete/Discrete Derivative  gainval=1.0  ICPrevScaledInput=0.0  OutMin=[]  OutMax=[]  OutDataType=fixdt(1, 16)  OutScaling=2^-10  DoSatur=off
  Discrete Derivative1 : simulink/Discrete/Discrete Derivative  gainval=1.0  ICPrevScaledInput=0.0  OutMin=[]  OutMax=[]  OutDataType=fixdt(1, 16)  OutScaling=2^-10  DoSatur=off
  Discrete Derivative2 : simulink/Discrete/Discrete Derivative  gainval=1.0  ICPrevScaledInput=0.0  OutMin=[]  OutMax=[]  OutDataType=fixdt(1, 16)  OutScaling=2^-10  DoSatur=off
  Discrete-Time Integrator4 : DiscreteIntegrator  SampleTime=1/1000  LimitOutput=on  UpperSaturationLimit=MC_YR_INT_LIM  LowerSaturationLimit=-MC_YR_INT_LIM  ICPrevOutput=DiscIntNeverNeededParam  ICPrevScaledInput=DiscIntNeverNeededParam
  Discrete-Time Integrator5 : DiscreteIntegrator  SampleTime=1/1000  LimitOutput=on  UpperSaturationLimit=MC_PR_INT_LIM  LowerSaturationLimit=-MC_PR_INT_LIM  ICPrevOutput=DiscIntNeverNeededParam  ICPrevScaledInput=DiscIntNeverNeededParam
  Discrete-Time Integrator6 : DiscreteIntegrator  SampleTime=1/1000  LimitOutput=on  UpperSaturationLimit=MC_RR_INT_LIM  LowerSaturationLimit=-MC_RR_INT_LIM  ICPrevOutput=DiscIntNeverNeededParam  ICPrevScaledInput=DiscIntNeverNeededParam
  Gain : Gain  Gain=MC_PITCHRATE_P
  Gain10 : Gain  Gain=MC_PITCHRATE_K
  Gain11 : Gain  Gain=MC_YAWRATE_K
  Gain12 : Gain  Gain=MC_ROLLRATE_K
  Gain13 : Gain  Gain=MC_YAWRATE_K
  Gain14 : Gain  Gain=MC_PITCHRATE_K
  Gain15 : Gain  Gain=MC_YAWRATE_I
  Gain16 : Gain  Gain=MC_PITCHRATE_I
  Gain17 : Gain  Gain=MC_ROLLRATE_I
  Gain2 : Gain  Gain=MC_PITCHRATE_D
  Gain3 : Gain  Gain=MC_YAWRATE_P
  Gain5 : Gain  Gain=MC_YAWRATE_D
  Gain6 : Gain  Gain=MC_ROLLRATE_P
  Gain8 : Gain  Gain=MC_ROLLRATE_D
  Gain9 : Gain  Gain=MC_ROLLRATE_K
  LTI System2 : cstblocks/LTI System  sys=c2d(tf(1,[IMU_GYRO_CUTOFF 1]),1/1000)  IC=[]  PadeOrder=0
  LTI System3 : cstblocks/LTI System  sys=c2d(tf(1,[IMU_GYRO_CUTOFF 1]),1/1000)  IC=[]  PadeOrder=0
  LTI System4 : cstblocks/LTI System  sys=c2d(tf(1,[IMU_GYRO_CUTOFF 1]),1/1000)  IC=[]  PadeOrder=0
  LTI System6 : cstblocks/LTI System  sys=c2d(tf(1,[IMU_DGYRO_CUTOFF 1]),1/1000)  IC=[]  PadeOrder=0
  Mux2 : Mux  Inputs=3
  PID Controller : slpidlib/PID Controller  Controller=I  Form=Parallel  TimeDomain=Discrete-time  UseExternalTs=off  SampleTime=1/1000  IntegratorMethod=Forward Euler  FilterMethod=Forward Euler  ControllerParametersSource=internal  P=1  I=MC_YAWRATE_I  UseKiTs=off  D=0  UseExternalDerivativeSource=off  N=100  UseFilter=on  TunerSelectOption=Transfer Function Based (PID Tuner App)  InitialConditionSource=internal  InitialConditionForIntegrator=0  InitialConditionForFilter=0  DifferentiatorICPrevScaledInput=0  ExternalReset=none  TrackingMode=off  Kt=1  LimitOutput=on  SatLimitsSource=internal  UpperSaturationLimit=MC_PR_INT_LIM  LowerSaturationLimit=-MC_PR_INT_LIM  LinearizeAsGain=off  AntiWindupMode=clamping  Kb=1  LimitIntegrator=off  UpperIntegratorSaturationLimit=inf  LowerIntegratorSaturationLimit=-inf  POutMin=[]  POutMax=[]  IOutMin=[]  IOutMax=[]  DOutMin=[]  DOutMax=[]  NOutMin=[]  NOutMax=[]  SumOutMin=[]  SumOutMax=[]  SaturationOutMin=[]  SaturationOutMax=[]  PParamMin=[]  PParamMax=[]  IParamMin=[]  IParamMax=[]  DParamMin=[]  DParamMax=[]  NParamMin=[]  NParamMax=[]  KbParamMin=[]  KbParamMax=[]  KtParamMin=[]  KtParamMax=[]  KbOutMin=[]  KbOutMax=[]  KtOutMin=[]  KtOutMax=[]  IntegratorOutMin=[]  IntegratorOutMax=[]  FilterOutMin=[]  FilterOutMax=[]  SumI1OutMin=[]  SumI1OutMax=[]  SumI2OutMin=[]  SumI2OutMax=[]  SumI3OutMin=[]  SumI3OutMax=[]  SumI4OutMin=[]  SumI4OutMax=[]  SumDOutMin=[]  SumDOutMax=[]  DifferentiatorOutMin=[]  DifferentiatorOutMax=[]  FilterDiffOutCoefMin=[]  FilterDiffOutCoefMax=[]  ReciprocalOutMin=[]  ReciprocalOutMax=[]  SumDenOutMin=[]  SumDenOutMax=[]  SumNumOutMin=[]  SumNumOutMax=[]  DivideOutMin=[]  DivideOutMax=[]  UdiffTsProdOutMin=[]  UdiffTsProdOutMax=[]  NTsProdOutMin=[]  NTsProdOutMax=[]  UintegralTsProdOutMin=[]  UintegralTsProdOutMax=[]  UngainTsProdOutMin=[]  UngainTsProdOutMax=[]  ClampingZeroOutDataTypeStr=Inherit: Inherit via back propagation  ClampingZeroOutMin=[]  ClampingZeroOutMax=[]  FilterDenConstantOutDataTypeStr=Inherit: Inherit via back propagation  FilterDenConstantOutMin=[]  FilterDenConstantOutMax=[]  PCopyOutDataTypeStr=Inherit: Inherit via back propagation  PCopyOutMin=[]  PCopyOutMax=[]  NCopyOutDataTypeStr=Inherit: Inherit via back propagation  NCopyOutMin=[]  NCopyOutMax=[]  IntegratorContinuousStateAttributes=''  IntegratorStateMustResolveToSignalObject=off  IntegratorRTWStateStorageClass=Auto  FilterContinuousStateAttributes=''  FilterStateMustResolveToSignalObject=off  FilterRTWStateStorageClass=Auto  ParallelPVariant=Disabled  IdealPVariant=Disabled  IVariant=InternalParameters  DVariant=Disabled  IntegratorVariant=Discrete  SatVariant=Enabled  AWVariant=DiscClampingParallel  PCopyVariant=Disabled  TRVariant=Disabled  FdbkBlocksVariant=Forward  IdealPFdbkVariant=Disabled  SatFdbkVariant=Disabled  DerivativeFilterVariant=Disabled  NVariant=Disabled  NCopyVariant=Disabled_SignalSpec  FilterICVariant=Disabled  IntegratorICVariant=InternalICs  ExternalResetVariant=Disabled  TRSumVariant=Passthrough  SumFdbkVariant=Disabled  SumVariant=Passthrough_I  TsampFilterVariant=InternalTs  TsampNgainVariant=Passthrough  TsampIntegralVariant=Disabled_SignalSpec  ExternalSaturationOutDataTypeStr=Inherit: Same as second input  DerivativeSourceVariant=Disabled
  PID Controller1 : slpidlib/PID Controller  Controller=I  Form=Parallel  TimeDomain=Discrete-time  UseExternalTs=off  SampleTime=1/1000  IntegratorMethod=Forward Euler  FilterMethod=Forward Euler  ControllerParametersSource=internal  P=1  I=MC_ROLLRATE_I  UseKiTs=off  D=0  UseExternalDerivativeSource=off  N=100  UseFilter=on  TunerSelectOption=Transfer Function Based (PID Tuner App)  InitialConditionSource=internal  InitialConditionForIntegrator=0  InitialConditionForFilter=0  DifferentiatorICPrevScaledInput=0  ExternalReset=none  TrackingMode=off  Kt=1  LimitOutput=on  SatLimitsSource=internal  UpperSaturationLimit=MC_RR_INT_LIM  LowerSaturationLimit=-MC_RR_INT_LIM  LinearizeAsGain=off  AntiWindupMode=clamping  Kb=1  LimitIntegrator=off  UpperIntegratorSaturationLimit=inf  LowerIntegratorSaturationLimit=-inf  POutMin=[]  POutMax=[]  IOutMin=[]  IOutMax=[]  DOutMin=[]  DOutMax=[]  NOutMin=[]  NOutMax=[]  SumOutMin=[]  SumOutMax=[]  SaturationOutMin=[]  SaturationOutMax=[]  PParamMin=[]  PParamMax=[]  IParamMin=[]  IParamMax=[]  DParamMin=[]  DParamMax=[]  NParamMin=[]  NParamMax=[]  KbParamMin=[]  KbParamMax=[]  KtParamMin=[]  KtParamMax=[]  KbOutMin=[]  KbOutMax=[]  KtOutMin=[]  KtOutMax=[]  IntegratorOutMin=[]  IntegratorOutMax=[]  FilterOutMin=[]  FilterOutMax=[]  SumI1OutMin=[]  SumI1OutMax=[]  SumI2OutMin=[]  SumI2OutMax=[]  SumI3OutMin=[]  SumI3OutMax=[]  SumI4OutMin=[]  SumI4OutMax=[]  SumDOutMin=[]  SumDOutMax=[]  DifferentiatorOutMin=[]  DifferentiatorOutMax=[]  FilterDiffOutCoefMin=[]  FilterDiffOutCoefMax=[]  ReciprocalOutMin=[]  ReciprocalOutMax=[]  SumDenOutMin=[]  SumDenOutMax=[]  SumNumOutMin=[]  SumNumOutMax=[]  DivideOutMin=[]  DivideOutMax=[]  UdiffTsProdOutMin=[]  UdiffTsProdOutMax=[]  NTsProdOutMin=[]  NTsProdOutMax=[]  UintegralTsProdOutMin=[]  UintegralTsProdOutMax=[]  UngainTsProdOutMin=[]  UngainTsProdOutMax=[]  ClampingZeroOutDataTypeStr=Inherit: Inherit via back propagation  ClampingZeroOutMin=[]  ClampingZeroOutMax=[]  FilterDenConstantOutDataTypeStr=Inherit: Inherit via back propagation  FilterDenConstantOutMin=[]  FilterDenConstantOutMax=[]  PCopyOutDataTypeStr=Inherit: Inherit via back propagation  PCopyOutMin=[]  PCopyOutMax=[]  NCopyOutDataTypeStr=Inherit: Inherit via back propagation  NCopyOutMin=[]  NCopyOutMax=[]  IntegratorContinuousStateAttributes=''  IntegratorStateMustResolveToSignalObject=off  IntegratorRTWStateStorageClass=Auto  FilterContinuousStateAttributes=''  FilterStateMustResolveToSignalObject=off  FilterRTWStateStorageClass=Auto  ParallelPVariant=Disabled  IdealPVariant=Disabled  IVariant=InternalParameters  DVariant=Disabled  IntegratorVariant=Discrete  SatVariant=Enabled  AWVariant=DiscClampingParallel  PCopyVariant=Disabled  TRVariant=Disabled  FdbkBlocksVariant=Forward  IdealPFdbkVariant=Disabled  SatFdbkVariant=Disabled  DerivativeFilterVariant=Disabled  NVariant=Disabled  NCopyVariant=Disabled_SignalSpec  FilterICVariant=Disabled  IntegratorICVariant=InternalICs  ExternalResetVariant=Disabled  TRSumVariant=Passthrough  SumFdbkVariant=Disabled  SumVariant=Passthrough_I  TsampFilterVariant=InternalTs  TsampNgainVariant=Passthrough  TsampIntegralVariant=Disabled_SignalSpec  ExternalSaturationOutDataTypeStr=Inherit: Same as second input  DerivativeSourceVariant=Disabled
  PID Controller2 : slpidlib/PID Controller  Controller=I  Form=Parallel  TimeDomain=Discrete-time  UseExternalTs=off  SampleTime=1/1000  IntegratorMethod=Forward Euler  FilterMethod=Forward Euler  ControllerParametersSource=internal  P=1  I=MC_PITCHRATE_I  UseKiTs=off  D=0  UseExternalDerivativeSource=off  N=100  UseFilter=on  TunerSelectOption=Transfer Function Based (PID Tuner App)  InitialConditionSource=internal  InitialConditionForIntegrator=0  InitialConditionForFilter=0  DifferentiatorICPrevScaledInput=0  ExternalReset=none  TrackingMode=off  Kt=1  LimitOutput=on  SatLimitsSource=internal  UpperSaturationLimit=MC_YR_INT_LIM  LowerSaturationLimit=-MC_YR_INT_LIM  LinearizeAsGain=off  AntiWindupMode=clamping  Kb=1  LimitIntegrator=off  UpperIntegratorSaturationLimit=inf  LowerIntegratorSaturationLimit=-inf  POutMin=[]  POutMax=[]  IOutMin=[]  IOutMax=[]  DOutMin=[]  DOutMax=[]  NOutMin=[]  NOutMax=[]  SumOutMin=[]  SumOutMax=[]  SaturationOutMin=[]  SaturationOutMax=[]  PParamMin=[]  PParamMax=[]  IParamMin=[]  IParamMax=[]  DParamMin=[]  DParamMax=[]  NParamMin=[]  NParamMax=[]  KbParamMin=[]  KbParamMax=[]  KtParamMin=[]  KtParamMax=[]  KbOutMin=[]  KbOutMax=[]  KtOutMin=[]  KtOutMax=[]  IntegratorOutMin=[]  IntegratorOutMax=[]  FilterOutMin=[]  FilterOutMax=[]  SumI1OutMin=[]  SumI1OutMax=[]  SumI2OutMin=[]  SumI2OutMax=[]  SumI3OutMin=[]  SumI3OutMax=[]  SumI4OutMin=[]  SumI4OutMax=[]  SumDOutMin=[]  SumDOutMax=[]  DifferentiatorOutMin=[]  DifferentiatorOutMax=[]  FilterDiffOutCoefMin=[]  FilterDiffOutCoefMax=[]  ReciprocalOutMin=[]  ReciprocalOutMax=[]  SumDenOutMin=[]  SumDenOutMax=[]  SumNumOutMin=[]  SumNumOutMax=[]  DivideOutMin=[]  DivideOutMax=[]  UdiffTsProdOutMin=[]  UdiffTsProdOutMax=[]  NTsProdOutMin=[]  NTsProdOutMax=[]  UintegralTsProdOutMin=[]  UintegralTsProdOutMax=[]  UngainTsProdOutMin=[]  UngainTsProdOutMax=[]  ClampingZeroOutDataTypeStr=Inherit: Inherit via back propagation  ClampingZeroOutMin=[]  ClampingZeroOutMax=[]  FilterDenConstantOutDataTypeStr=Inherit: Inherit via back propagation  FilterDenConstantOutMin=[]  FilterDenConstantOutMax=[]  PCopyOutDataTypeStr=Inherit: Inherit via back propagation  PCopyOutMin=[]  PCopyOutMax=[]  NCopyOutDataTypeStr=Inherit: Inherit via back propagation  NCopyOutMin=[]  NCopyOutMax=[]  IntegratorContinuousStateAttributes=''  IntegratorStateMustResolveToSignalObject=off  IntegratorRTWStateStorageClass=Auto  FilterContinuousStateAttributes=''  FilterStateMustResolveToSignalObject=off  FilterRTWStateStorageClass=Auto  ParallelPVariant=Disabled  IdealPVariant=Disabled  IVariant=InternalParameters  DVariant=Disabled  IntegratorVariant=Discrete  SatVariant=Enabled  AWVariant=DiscClampingParallel  PCopyVariant=Disabled  TRVariant=Disabled  FdbkBlocksVariant=Forward  IdealPFdbkVariant=Disabled  SatFdbkVariant=Disabled  DerivativeFilterVariant=Disabled  NVariant=Disabled  NCopyVariant=Disabled_SignalSpec  FilterICVariant=Disabled  IntegratorICVariant=InternalICs  ExternalResetVariant=Disabled  TRSumVariant=Passthrough  SumFdbkVariant=Disabled  SumVariant=Passthrough_I  TsampFilterVariant=InternalTs  TsampNgainVariant=Passthrough  TsampIntegralVariant=Disabled_SignalSpec  ExternalSaturationOutDataTypeStr=Inherit: Same as second input  DerivativeSourceVariant=Disabled
  PID Controller3 : slpidlib/PID Controller  Controller=PID  Form=Parallel  TimeDomain=Continuous-time  UseExternalTs=off  SampleTime=-1  IntegratorMethod=Forward Euler  FilterMethod=Forward Euler  ControllerParametersSource=internal  P=1  I=1  UseKiTs=off  D=0  UseExternalDerivativeSource=off  N=100  UseFilter=on  TunerSelectOption=Transfer Function Based (PID Tuner App)  InitialConditionSource=internal  InitialConditionForIntegrator=0  InitialConditionForFilter=0  DifferentiatorICPrevScaledInput=0  ExternalReset=none  TrackingMode=off  Kt=1  LimitOutput=off  SatLimitsSource=internal  UpperSaturationLimit=inf  LowerSaturationLimit=-inf  LinearizeAsGain=on  AntiWindupMode=none  Kb=1  LimitIntegrator=off  UpperIntegratorSaturationLimit=inf  LowerIntegratorSaturationLimit=-inf  POutMin=[]  POutMax=[]  IOutMin=[]  IOutMax=[]  DOutMin=[]  DOutMax=[]  NOutMin=[]  NOutMax=[]  SumOutMin=[]  SumOutMax=[]  SaturationOutMin=[]  SaturationOutMax=[]  PParamMin=[]  PParamMax=[]  IParamMin=[]  IParamMax=[]  DParamMin=[]  DParamMax=[]  NParamMin=[]  NParamMax=[]  KbParamMin=[]  KbParamMax=[]  KtParamMin=[]  KtParamMax=[]  KbOutMin=[]  KbOutMax=[]  KtOutMin=[]  KtOutMax=[]  IntegratorOutMin=[]  IntegratorOutMax=[]  FilterOutMin=[]  FilterOutMax=[]  SumI1OutMin=[]  SumI1OutMax=[]  SumI2OutMin=[]  SumI2OutMax=[]  SumI3OutMin=[]  SumI3OutMax=[]  SumI4OutMin=[]  SumI4OutMax=[]  SumDOutMin=[]  SumDOutMax=[]  DifferentiatorOutMin=[]  DifferentiatorOutMax=[]  FilterDiffOutCoefMin=[]  FilterDiffOutCoefMax=[]  ReciprocalOutMin=[]  ReciprocalOutMax=[]  SumDenOutMin=[]  SumDenOutMax=[]  SumNumOutMin=[]  SumNumOutMax=[]  DivideOutMin=[]  DivideOutMax=[]  UdiffTsProdOutMin=[]  UdiffTsProdOutMax=[]  NTsProdOutMin=[]  NTsProdOutMax=[]  UintegralTsProdOutMin=[]  UintegralTsProdOutMax=[]  UngainTsProdOutMin=[]  UngainTsProdOutMax=[]  ClampingZeroOutDataTypeStr=Inherit: Inherit via back propagation  ClampingZeroOutMin=[]  ClampingZeroOutMax=[]  FilterDenConstantOutDataTypeStr=Inherit: Inherit via back propagation  FilterDenConstantOutMin=[]  FilterDenConstantOutMax=[]  PCopyOutDataTypeStr=Inherit: Inherit via back propagation  PCopyOutMin=[]  PCopyOutMax=[]  NCopyOutDataTypeStr=Inherit: Inherit via back propagation  NCopyOutMin=[]  NCopyOutMax=[]  IntegratorContinuousStateAttributes=''  IntegratorStateMustResolveToSignalObject=off  IntegratorRTWStateStorageClass=Auto  FilterContinuousStateAttributes=''  FilterStateMustResolveToSignalObject=off  FilterRTWStateStorageClass=Auto  ParallelPVariant=InternalParameters  IdealPVariant=Disabled  IVariant=InternalParameters  DVariant=InternalParameters  IntegratorVariant=Continuous  SatVariant=Disabled  AWVariant=Passthrough  PCopyVariant=Disabled  TRVariant=Disabled  FdbkBlocksVariant=Forward  IdealPFdbkVariant=Disabled  SatFdbkVariant=Disabled  DerivativeFilterVariant=ContFilter  NVariant=InternalParameters  NCopyVariant=Disabled  FilterICVariant=InternalICsFilter  IntegratorICVariant=InternalICs  ExternalResetVariant=Disabled  TRSumVariant=Passthrough  SumFdbkVariant=Disabled  SumVariant=Sum_PID  TsampFilterVariant=InternalTs  TsampNgainVariant=Passthrough  TsampIntegralVariant=Disabled_SignalSpec  ExternalSaturationOutDataTypeStr=Inherit: Same as second input  DerivativeSourceVariant=ErrorSignal
  Sum : Sum  Inputs=|+-
  Sum1 : Sum  Inputs=|+-
  Sum2 : Sum  Inputs=|+-
  Delta S.P : Outport
  wires:
  Sum/1 -> Gain10/1
  Gain2/1 -> Add/3
  Gain10/1 -> PID Controller/1, Gain/1
  Gain/1 -> Add/1
  Gain3/1 -> Add1/1
  Gain5/1 -> Add1/3
  Sum1/1 -> Gain11/1
  [dPsi] -> Gain13/1, Sum1/2  "Feedback"
  [SP_dPsi] -> Sum1/1  "Setpoint"
  Add/1 -> Mux2/2
  Mux2/1 -> Delta S.P/1
  Gain6/1 -> Add2/1
  Gain9/1 -> PID Controller1/1, Gain6/1
  Gain8/1 -> Add2/3
  Sum2/1 -> Gain9/1
  [SP_dPhi] -> Sum2/1  "Setpoint"
  [SP_dTheta] -> Sum/1  "Setpoint"
  [Phi] -> Gain12/1, Sum2/2  "Feedback"
  [Theta] -> Gain14/1, Sum/2  "Feedback"
  Add1/1 -> Mux2/3
  Discrete Derivative/1 -> Gain8/1
  Discrete Derivative1/1 -> Gain2/1
  Discrete Derivative2/1 -> Gain5/1
  Gyro/1 -> Demux/1
  Add2/1 -> Mux2/1
  rates s.p/1 -> Demux1/1
  Demux1/1 -> [SP_dPhi]
  Demux1/2 -> [SP_dTheta]
  Demux1/3 -> [SP_dPsi]
  Demux/3 -> [dPsi]
  Demux/1 -> [Phi]
  Demux/2 -> [Theta]
  Gain12/1 -> Discrete Derivative/1
  Gain14/1 -> Discrete Derivative1/1
  Gain13/1 -> Discrete Derivative2/1
  Gain11/1 -> PID Controller2/1, Gain3/1
  PID Controller2/1 -> Add1/2
  PID Controller/1 -> Add/2
  PID Controller1/1 -> Add2/2

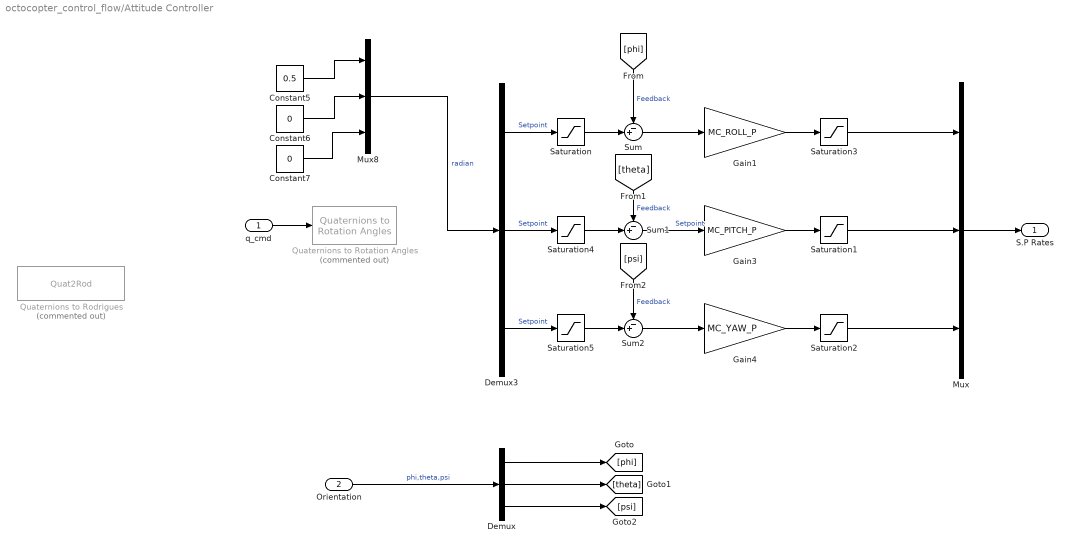
== system octocopter_control_flow/Attitude Controller ==
  q_cmd : Inport
  Orientation : Inport  Port=2
  Constant5 : Constant  Value=0.5
  Constant6 : Constant  Value=0
  Constant7 : Constant  Value=0
  Demux : Demux  Outputs=3
  Demux3 : Demux  Outputs=3
  Gain1 : Gain  Gain=MC_ROLL_P
  Gain3 : Gain  Gain=MC_PITCH_P
  Gain4 : Gain  Gain=MC_YAW_P
  Mux : Mux  Inputs=3
  Mux8 : Mux  Inputs=3
  Quaternions to Rodrigues : Quat2Rod  Commented=on
  Quaternions to Rotation Angles : sharedtransform/Quaternions to Rotation Angles  Commented=on  rotationOrder=XYZ  aMode=aMode
  Saturation : Saturate  UpperLimit=pi/2  LowerLimit=-pi/2
  Saturation1 : Saturate  UpperLimit=MC_PITCHRATE_MAX  LowerLimit=-MC_PITCHRATE_MAX
  Saturation2 : Saturate  UpperLimit=MC_YAWRATE_MAX  LowerLimit=-MC_YAWRATE_MAX
  Saturation3 : Saturate  UpperLimit=MC_ROLLRATE_MAX  LowerLimit=-MC_ROLLRATE_MAX
  Saturation4 : Saturate  UpperLimit=pi/2  LowerLimit=-pi/2
  Saturation5 : Saturate  UpperLimit=+pi  LowerLimit=-pi
  Sum : Sum  Inputs=-+|
  Sum1 : Sum  Inputs=-+|
  Sum2 : Sum  Inputs=-+|
  S.P Rates : Outport
  wires:
  Orientation/1 -> Demux/1  "phi,theta,psi"
  Demux/2 -> [theta]
  Demux/1 -> [phi]
  Demux/3 -> [psi]
  Demux3/1 -> Saturation/1  "Setpoint"
  Demux3/2 -> Saturation4/1  "Setpoint"
  Demux3/3 -> Saturation5/1  "Setpoint"
  Gain1/1 -> Saturation3/1
  Gain3/1 -> Saturation1/1
  Gain4/1 -> Saturation2/1
  Saturation1/1 -> Mux/2
  Saturation2/1 -> Mux/3
  [phi] -> Sum/1  "Feedback"
  Sum/1 -> Gain1/1
  [theta] -> Sum1/1  "Feedback"
  Sum2/1 -> Gain4/1
  [psi] -> Sum2/1  "Feedback"
  Sum1/1 -> Gain3/1  "Setpoint"
  q_cmd/1 -> Quaternions to Rotation Angles/1
  Saturation/1 -> Sum/2
  Saturation4/1 -> Sum1/2
  Saturation5/1 -> Sum2/2
  Saturation3/1 -> Mux/1
  Mux/1 -> S.P Rates/1
  Constant5/1 -> Mux8/1
  Constant7/1 -> Mux8/3
  Constant6/1 -> Mux8/2
  Mux8/1 -> Demux3/1  "radian"

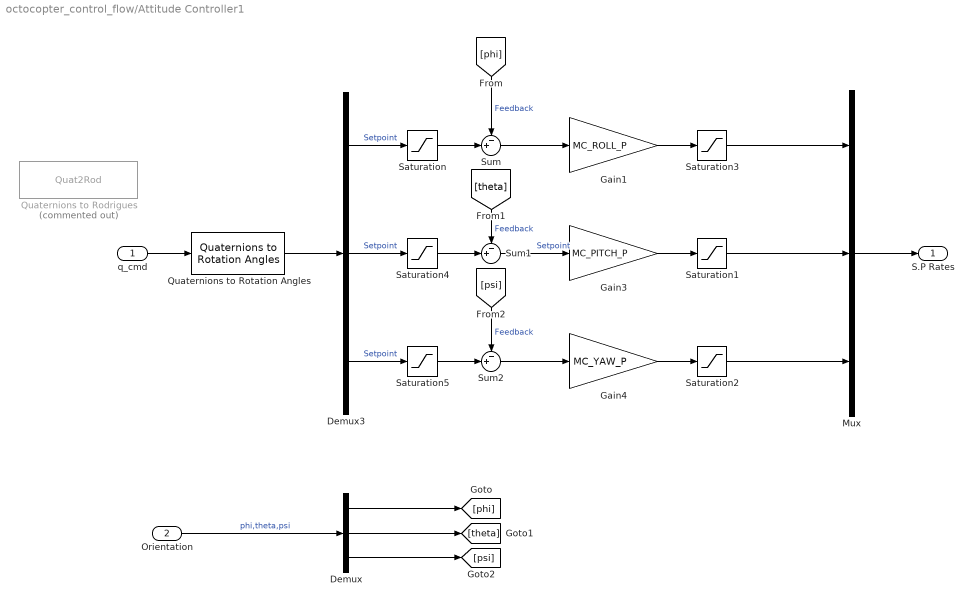
== system octocopter_control_flow/Attitude Controller1 ==
  q_cmd : Inport
  Orientation : Inport  Port=2
  Demux : Demux  Outputs=3
  Demux3 : Demux  Outputs=3
  Gain1 : Gain  Gain=MC_ROLL_P
  Gain3 : Gain  Gain=MC_PITCH_P
  Gain4 : Gain  Gain=MC_YAW_P
  Mux : Mux  Inputs=3
  Quaternions to Rodrigues : Quat2Rod  Commented=on
  Quaternions to Rotation Angles : sharedtransform/Quaternions to Rotation Angles  rotationOrder=XYZ  aMode=aMode
  Saturation : Saturate  UpperLimit=pi/2  LowerLimit=-pi/2
  Saturation1 : Saturate  UpperLimit=MC_PITCHRATE_MAX  LowerLimit=-MC_PITCHRATE_MAX
  Saturation2 : Saturate  UpperLimit=MC_YAWRATE_MAX  LowerLimit=-MC_YAWRATE_MAX
  Saturation3 : Saturate  UpperLimit=MC_ROLLRATE_MAX  LowerLimit=-MC_ROLLRATE_MAX
  Saturation4 : Saturate  UpperLimit=pi/2  LowerLimit=-pi/2
  Saturation5 : Saturate  UpperLimit=+pi  LowerLimit=-pi
  Sum : Sum  Inputs=-+|
  Sum1 : Sum  Inputs=-+|
  Sum2 : Sum  Inputs=-+|
  S.P Rates : Outport
  wires:
  Mux/1 -> S.P Rates/1
  Saturation3/1 -> Mux/1
  Saturation5/1 -> Sum2/2
  Saturation4/1 -> Sum1/2
  Saturation/1 -> Sum/2
  Quaternions to Rotation Angles/1 -> Demux3/1
  q_cmd/1 -> Quaternions to Rotation Angles/1
  Sum1/1 -> Gain3/1  "Setpoint"
  [psi] -> Sum2/1  "Feedback"
  Sum2/1 -> Gain4/1
  [theta] -> Sum1/1  "Feedback"
  Sum/1 -> Gain1/1
  [phi] -> Sum/1  "Feedback"
  Saturation2/1 -> Mux/3
  Saturation1/1 -> Mux/2
  Gain4/1 -> Saturation2/1
  Gain3/1 -> Saturation1/1
  Gain1/1 -> Saturation3/1
  Demux3/3 -> Saturation5/1  "Setpoint"
  Demux3/2 -> Saturation4/1  "Setpoint"
  Demux3/1 -> Saturation/1  "Setpoint"
  Demux/3 -> [psi]
  Demux/1 -> [phi]
  Demux/2 -> [theta]
  Orientation/1 -> Demux/1  "phi,theta,psi"

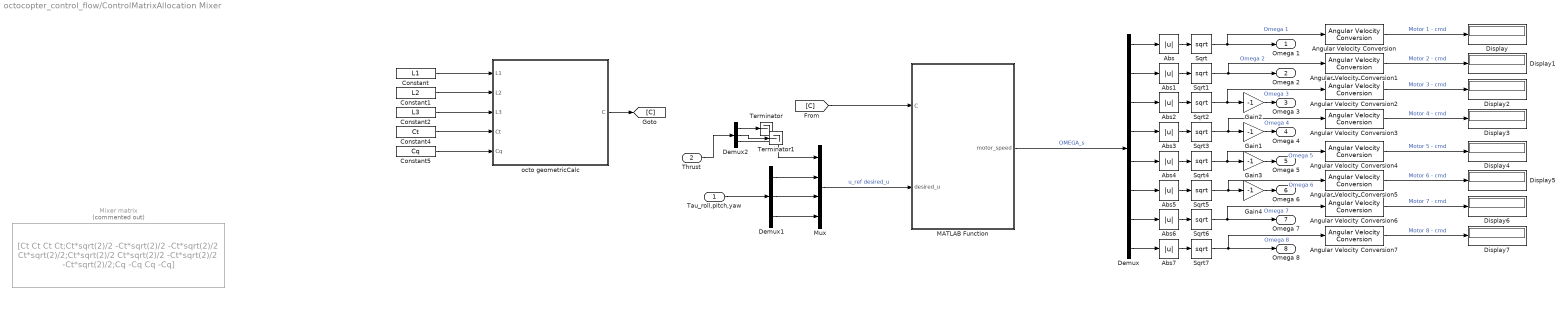
== system octocopter_control_flow/ControlMatrixAllocation Mixer ==
  Tau_roll,pitch,yaw : Inport
  Thrust : Inport  Port=2
  Abs{,1..7} (8 alike) : Abs  SaturateOnIntegerOverflow=off
  Angular Velocity Conversion{,1..7} (8 alike) : aerolibconvert2/Angular Velocity Conversion  IU=rad/s  OU=rpm
  Constant : Constant  Value=L1
  Constant1 : Constant  Value=L2
  Constant2 : Constant  Value=L3
  Constant4 : Constant  Value=Ct
  Constant5 : Constant  Value=Cq
  Demux : Demux  Outputs=8
  Demux1 : Demux  Outputs=3
  Demux2 : Demux  Outputs=3
  Display{,1..7} (8 alike) : Display
  Gain{1..4} (4 alike) : Gain  Gain=-1
  MATLAB Function : MATLAB Function  TreatAsAtomicUnit=on
  Mixer matrix : Constant  Commented=on  StartFcn=|  Value=[Ct Ct Ct Ct;Ct*sqrt(2)/2 -Ct*sqrt(2)/2 -Ct*sqrt(2)/2 Ct*sqrt(2)/2;Ct*sqrt(2)/2 Ct*sqrt(2)/2 -Ct*sqrt(2)/2 -Ct*sqrt(2)/2;Cq -Cq Cq -Cq]  OutDataTypeStr=Inherit: Inherit via back propagation  SampleTime=1/1000
      | %p = Simulink.Mask.get('ControlsModels/Moments and Forces');
      | 
      | Ct = 0.025
      | Cq = 2e-6;
      | 
      | %Ct = p.getParameter('Ct');
      | %Cq =p.getParameter('Cq');
      | 
      | %Ct = str2double(Ct.Value);
      | %Cq = str2double(Cq.Value);
  Mux : Mux
  Sqrt{,1..7} (8 alike) : Sqrt
  Terminator : Terminator
  Terminator1 : Terminator
  octo geometricCalc : MATLAB Function  TreatAsAtomicUnit=on
  Omega 1 : Outport
  Omega 2 : Outport  Port=2
  Omega 3 : Outport  Port=3
  Omega 4 : Outport  Port=4
  Omega 5 : Outport  Port=5
  Omega 6 : Outport  Port=6
  Omega 7 : Outport  Port=7
  Omega 8 : Outport  Port=8
  wires:
  Demux/1 -> Abs/1
  Demux/2 -> Abs1/1
  Demux/3 -> Abs2/1
  Demux/4 -> Abs3/1
  MATLAB Function/1(motor_speed) -> Demux/1  "OMEGA_s"
  Mux/1 -> MATLAB Function/2(desired_u)  "u_ref desired_u"
  Sqrt/1 -> Omega 1/1, Angular Velocity Conversion/1  "Omega 1"
  Sqrt1/1 -> Omega 2/1, Angular Velocity Conversion1/1  "Omega 2"
  Sqrt2/1 -> Gain2/1, Angular Velocity Conversion2/1  "Omega 3"
  Sqrt3/1 -> Gain1/1, Angular Velocity Conversion3/1  "Omega 4"
  Tau_roll,pitch,yaw/1 -> Demux1/1
  Demux1/3 -> Mux/4
  Demux1/1 -> Mux/2
  Demux1/2 -> Mux/3
  Angular Velocity Conversion/1 -> Display/1  "Motor 1 - cmd"
  Angular Velocity Conversion1/1 -> Display1/1  "Motor 2 - cmd"
  Angular Velocity Conversion2/1 -> Display2/1  "Motor 3 - cmd"
  Angular Velocity Conversion3/1 -> Display3/1  "Motor 4 - cmd"
  Abs/1 -> Sqrt/1
  Abs1/1 -> Sqrt1/1
  Abs2/1 -> Sqrt2/1
  Abs3/1 -> Sqrt3/1
  Gain1/1 -> Omega 4/1
  Constant1/1 -> octo geometricCalc/2(L2)
  Constant/1 -> octo geometricCalc/1(L1)
  octo geometricCalc/1(C) -> [C]
  Constant2/1 -> octo geometricCalc/3(L3)
  [C] -> MATLAB Function/1(C)
  Constant4/1 -> octo geometricCalc/4(Ct)
  Constant5/1 -> octo geometricCalc/5(Cq)
  Abs7/1 -> Sqrt7/1
  Demux/7 -> Abs6/1
  Angular Velocity Conversion5/1 -> Display5/1  "Motor 6 - cmd"
  Demux/5 -> Abs4/1
  Angular Velocity Conversion7/1 -> Display7/1  "Motor 8 - cmd"
  Sqrt5/1 -> Gain4/1, Angular Velocity Conversion5/1  "Omega 6"
  Angular Velocity Conversion4/1 -> Display4/1  "Motor 5 - cmd"
  Demux/6 -> Abs5/1
  Sqrt4/1 -> Gain3/1, Angular Velocity Conversion4/1  "Omega 5"
  Abs4/1 -> Sqrt4/1
  Abs6/1 -> Sqrt6/1
  Demux/8 -> Abs7/1
  Gain4/1 -> Omega 6/1
  Sqrt6/1 -> Omega 7/1, Angular Velocity Conversion6/1  "Omega 7"
  Angular Velocity Conversion6/1 -> Display6/1  "Motor 7 - cmd"
  Abs5/1 -> Sqrt5/1
  Sqrt7/1 -> Omega 8/1, Angular Velocity Conversion7/1  "Omega 8"
  Thrust/1 -> Demux2/1
  Demux2/3 -> Mux/1
  Demux2/1 -> Terminator/1
  Demux2/2 -> Terminator1/1
  Gain2/1 -> Omega 3/1
  Gain3/1 -> Omega 5/1

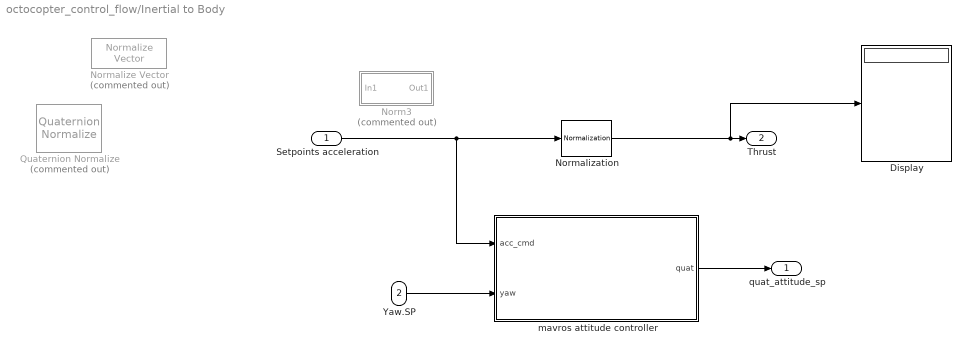
== system octocopter_control_flow/Inertial to Body ==
  Setpoints acceleration : Inport
  Yaw.SP : Inport  Port=2
  Display : Display
  Norm3 : Subsystem  Commented=on
      mask Display: disp('Norm')
  Normalization : dspmathops/Normalization  NormType=Squared 2-norm  Bias=1e-10  NormOver=Each column  Dimension=1  roundingMode=Floor  overflowMode=off  accumDataTypeStr=Inherit: Same as product output  accumLastDataTypeStr=Inherit: Same as product output  outputDataTypeStr=Inherit: Same as product output  outputMin=[]  outputMax=[]  outputLastDataTypeStr=Inherit: Same as product output
  Normalize Vector : vrlib/Utilities/Normalize Vector  Commented=on  maxzero=0
  Quaternion Normalize : sharedutil/Quaternion Normalize  Commented=on  aMode=aMode
  mavros attitude controller : Subsystem
      mask Display:
      | disp('Mavros Geometric controller')
      | port_label('input',1,'acc_{cmd}','texmode','on')
      | port_label('input',2,'\psi_{cmd}','texmode','on')
      | 
      | 
      | port_label('output',1,'quat','texmode','on')
  quat_attitude_sp : Outport
  Thrust : Outport  Port=2
  wires:
  Normalization/1 -> Display/1, Thrust/1
  Yaw.SP/1 -> mavros attitude controller/2(yaw)
  mavros attitude controller/1(quat) -> quat_attitude_sp/1
  Setpoints acceleration/1 -> Normalization/1, mavros attitude controller/1(acc_cmd)

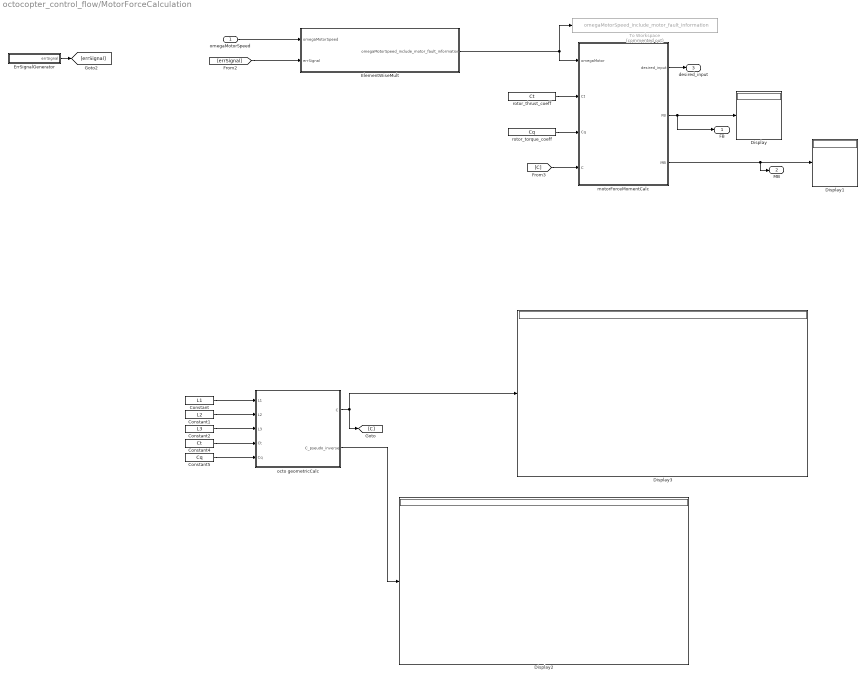
== system octocopter_control_flow/MotorForceCalculation ==
  omegaMotorSpeed : Inport
  Constant : Constant  Value=L1
  Constant1 : Constant  Value=L2
  Constant2 : Constant  Value=L3
  Constant4 : Constant  Value=Ct
  Constant5 : Constant  Value=Cq
  Display{,1..3} (4 alike) : Display
  ElementWiseMult : MATLAB Function  TreatAsAtomicUnit=on
  ErrSignalGenerator : Subsystem
  To Workspace : ToWorkspace  Commented=on  VariableName=omegaMotorSpeed_include_motor_fault_information  SampleTime=-1
  motorForceMomentCalc : MATLAB Function  TreatAsAtomicUnit=on
  octo geometricCalc : MATLAB Function  TreatAsAtomicUnit=on
  rotor_thrust_coeff : Constant  Value=Ct
  rotor_torque_coeff : Constant  Value=Cq
  FB : Outport
  MB : Outport  Port=2
  desired_input : Outport  Port=3
  wires:
  motorForceMomentCalc/2(FB) -> Display/1, FB/1
  motorForceMomentCalc/3(MB) -> Display1/1, MB/1
  rotor_thrust_coeff/1 -> motorForceMomentCalc/2(Ct)
  rotor_torque_coeff/1 -> motorForceMomentCalc/3(Cq)
  omegaMotorSpeed/1 -> ElementWiseMult/1(omegaMotorSpeed)
  ErrSignalGenerator/1(errSignal) -> [errSignal]
  [errSignal] -> ElementWiseMult/2(errSignal)
  ElementWiseMult/1(omegaMotorSpeed_include_motor_fault_information) -> motorForceMomentCalc/1(omegaMotor), To Workspace/1
  [C] -> motorForceMomentCalc/4(C)
  motorForceMomentCalc/1(desired_input) -> desired_input/1
  Constant2/1 -> octo geometricCalc/3(L3)
  Constant5/1 -> octo geometricCalc/5(Cq)
  Constant/1 -> octo geometricCalc/1(L1)
  Constant4/1 -> octo geometricCalc/4(Ct)
  octo geometricCalc/1(C) -> [C], Display3/1
  Constant1/1 -> octo geometricCalc/2(L2)
  octo geometricCalc/2(C_pseudo_inverse) -> Display2/1
